simulink model "Final_project_316_thirdl"  (R2014b)
settings: Solver=ode45  StartTime=0.0  StopTime=200  RelTol=1e-3
libraries: simulink x1
settings Model: Creator=Mike  LastModifiedBy=Mike

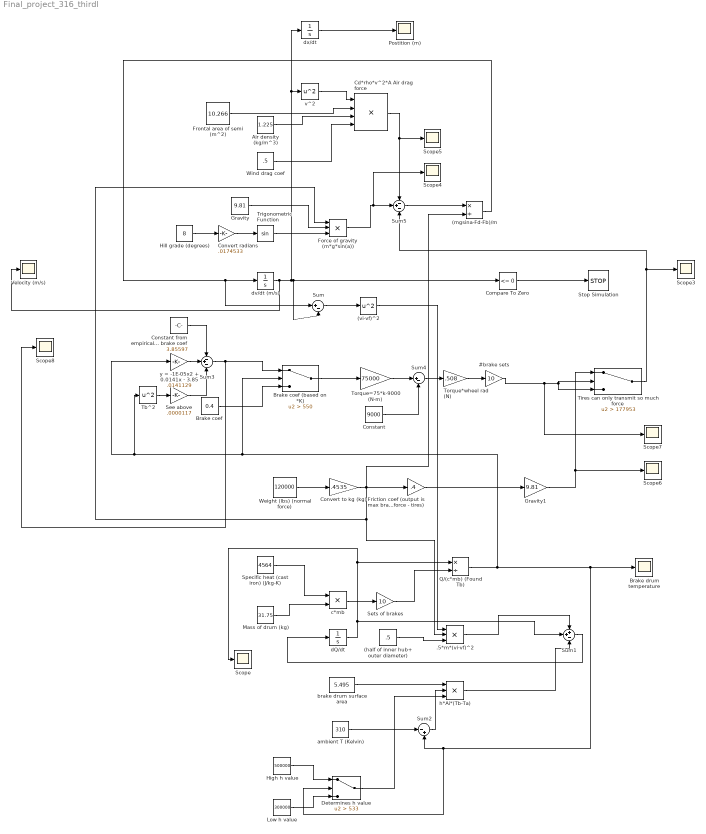
== system Final_project_316_thirdl ==
  #brake sets : Gain  Gain=10
  (half of inner hub+ outer diameter) : Constant  Value=.5
  (mgsina-Fd-Fb)/m : Product  Inputs=*/
  (vi-vf)^2 : Math  Operator=square  SaturateOnIntegerOverflow=on
  .5*m*(vi-vf)^2 : Product  Inputs=3
  Air density (kg/m^3) : Constant  Value=1.225
  Brake coef : Constant  Value=0.4
  Brake coef (based on *K) : Switch  Criteria=u2 > Threshold  Threshold=550
  Brake drum temperature : Scope
      settings: YMin=30  YMax=50  SaveName=ScopeData2
  Cd*rho*v^2*A Air drag force : Product  Inputs=4
  Compare To Zero : simulink/Logic and Bit Operations/Compare To Zero  relop=<=  OutDataTypeStr=boolean
  Constant : Constant  Value=9000
  Constant from empirical temp vs brake coef : Constant  Value=3.85597
  Convert radians : Gain  Gain=.0174533
  Convert to kg (kg) : Gain  Gain=.4535
  Determines h value : Switch  Criteria=u2 > Threshold  Threshold=533  ZeroCross=off
  Force of gravity (m*g*sin(a)) : Product  Inputs=3
  Friction coef (output is max brake force - tires) : Gain  Gain=.4
  Frontal area of semi (m^2) : Constant  Value=10.266
  Gravity : Constant  Value=9.81
  "Gravity1 " : Gain  Gain=9.81
  High h value : Constant  Value=500000
  Hill grade (degrees) : Constant  Value=8
  Low h value : Constant  Value=300000
  Mass of drum (kg) : Constant  Value=31.75
  Postition (m) : Scope
      settings: SaveName=ScopeData3
  Q/(c*mb) (Found Tb) : Product  Inputs=*/
  Scope{,3..8} (7 alike) : Scope
      Scope3 settings: SaveName=ScopeData4
      Scope4 settings: SaveName=ScopeData5
      Scope5 settings: SaveName=ScopeData6
      Scope6 settings: SaveName=ScopeData7
      Scope7 settings: SaveName=ScopeData8
      Scope8 settings: SaveName=ScopeData9
  "See above " : Gain  Gain=.0000117
  Sets of brakes : Gain  Gain=10
  Specific heat (cast iron) (J/kg-K) : Constant  Value=4564
  Stop Simulation : Stop
  Sum : Sum  Inputs=|+-
  Sum1 : Sum  Inputs=++-
  Sum2 : Sum  Inputs=|-+
  Sum3 : Sum  Inputs=-+-
  Sum4 : Sum  Inputs=|+-
  Sum5 : Sum  Inputs=-+-
  Tb^2 : Math  Operator=square  SaturateOnIntegerOverflow=on
  Tires can only transmit so much force : Switch  Criteria=u2 > Threshold  Threshold=177953
  Torque*wheel rad (N) : Gain  Gain=.508
  Torque=75*k-9000 (N-m) : Gain  Gain=75000
  Trigonometric Function : Trigonometry
  Velocity (m/s) : Scope
      settings: TimeRange=200
  Weight (lbs) (normal force) : Constant  Value=120000
  Wind drag coef : Constant  Value=.5
  ambient T (Kelvin) : Constant  Value=310
  brake drum surface area : Constant  Value=5.495
  c*mb : Product
  dQ/dt : Integrator  InitialCondition=1
  dv/dt (m/s) : Integrator  InitialCondition=24.3
  dx/dt : Integrator
  h*Ai*(Tb-Ta) : Product  Inputs=3
  v^2 : Math  Operator=square  SaturateOnIntegerOverflow=on
  "y = -1E-05x2 + 0.0141x - 3.85 " : Gain  Gain=.0141129
  wires:
  Weight (lbs) (normal force)/1 -> Convert to kg (kg)/1
  dQ/dt/1 -> Sum1/2, Scope/1, Q/(c*mb) (Found Tb)/1
  (half of inner hub+ outer diameter)/1 -> .5*m*(vi-vf)^2/3
  Convert to kg (kg)/1 -> (mgsina-Fd-Fb)/m/2, Force of gravity (m*g*sin(a))/1, .5*m*(vi-vf)^2/2, Friction coef (output is max brake force - tires)/1
  dv/dt (m/s)/1 -> Velocity (m/s)/1, dx/dt/1, v^2/1, Compare To Zero/1, Sum/2
  (mgsina-Fd-Fb)/m/1 -> dv/dt (m/s)/1, Sum/1
  Sum/1 -> (vi-vf)^2/1
  (vi-vf)^2/1 -> .5*m*(vi-vf)^2/1
  Sum1/1 -> dQ/dt/1
  brake drum surface area/1 -> h*Ai*(Tb-Ta)/1
  h*Ai*(Tb-Ta)/1 -> Sum1/3
  ambient T (Kelvin)/1 -> Sum2/1
  Specific heat (cast iron) (J/kg-K)/1 -> c*mb/1
  Mass of drum (kg)/1 -> c*mb/2
  c*mb/1 -> Sets of brakes/1
  Sets of brakes/1 -> Q/(c*mb) (Found Tb)/2
  Q/(c*mb) (Found Tb)/1 -> "y = -1E-05x2 + 0.0141x - 3.85 "/1, Tb^2/1, Brake coef (based on *K)/2, Brake drum temperature/1, Determines h value/2, Sum2/2
  Sum2/1 -> h*Ai*(Tb-Ta)/2
  Low h value/1 -> Determines h value/3
  High h value/1 -> Determines h value/1
  Determines h value/1 -> h*Ai*(Tb-Ta)/3
  Brake coef/1 -> Brake coef (based on *K)/3
  Sum3/1 -> Brake coef (based on *K)/1, Scope8/1
  Constant from empirical temp vs brake coef/1 -> Sum3/1
  "y = -1E-05x2 + 0.0141x - 3.85 "/1 -> Sum3/2
  "See above "/1 -> Sum3/3
  Tb^2/1 -> "See above "/1
  Brake coef (based on *K)/1 -> Torque=75*k-9000 (N-m)/1
  Torque=75*k-9000 (N-m)/1 -> Sum4/1
  Constant/1 -> Sum4/2
  Sum4/1 -> Torque*wheel rad (N)/1
  Torque*wheel rad (N)/1 -> #brake sets/1
  #brake sets/1 -> Scope7/1, Tires can only transmit so much force/3, Tires can only transmit so much force/2
  Force of gravity (m*g*sin(a))/1 -> Scope4/1, Sum5/2
  Gravity/1 -> Force of gravity (m*g*sin(a))/2
  Hill grade (degrees)/1 -> Convert radians/1
  Convert radians/1 -> Trigonometric Function/1
  Trigonometric Function/1 -> Force of gravity (m*g*sin(a))/3
  Wind drag coef/1 -> Cd*rho*v^2*A Air drag force/4
  Air density (kg/m^3)/1 -> Cd*rho*v^2*A Air drag force/3
  Frontal area of semi (m^2)/1 -> Cd*rho*v^2*A Air drag force/2
  v^2/1 -> Cd*rho*v^2*A Air drag force/1
  Cd*rho*v^2*A Air drag force/1 -> Scope5/1, Sum5/1
  Sum5/1 -> (mgsina-Fd-Fb)/m/1
  Friction coef (output is max brake force - tires)/1 -> "Gravity1 "/1
  .5*m*(vi-vf)^2/1 -> Sum1/1
  Compare To Zero/1 -> Stop Simulation/1
  dx/dt/1 -> Postition (m)/1
  Tires can only transmit so much force/1 -> Scope3/1, Sum5/3
  "Gravity1 "/1 -> Scope6/1, Tires can only transmit so much force/1
